simulink model "gm_sampleModel1668_5_sub_sub_sub"  (R2023a)
settings: Solver=VariableStepAuto  StartTime=0.0  StopTime=10.0  RelTol=1e-3
libraries: hdlsllib x7, simulink x1
settings Model: Creator=user1  LastModifiedBy=user1
settings OptimizationCC: BlockReduction=off  ConditionallyExecuteInputs=off
settings DebuggingCC: InheritedTsInSrcMsg=none

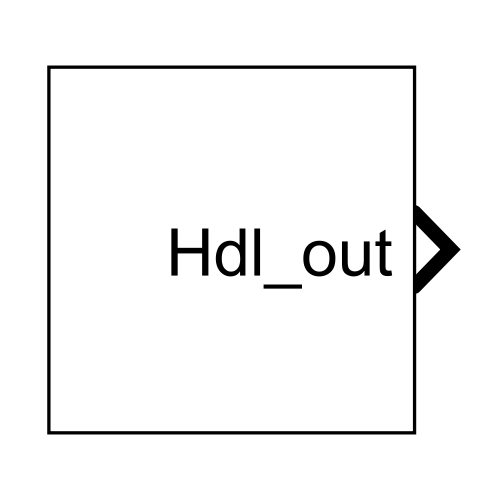
[thumbnail: Simulink's stored preview of the top-level diagram]
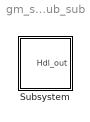
== system gm_sampleModel1668_5_sub_sub_sub ==
  Subsystem : Subsystem

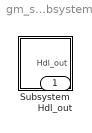
== system gm_sampleModel1668_5_sub_sub_sub/Subsystem ==
  Subsystem : Subsystem
  Hdl_out : Outport  OutDataTypeStr=uint8

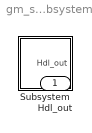
== system gm_sampleModel1668_5_sub_sub_sub/Subsystem/Subsystem ==
  Subsystem : Subsystem
  Hdl_out : Outport  OutDataTypeStr=uint8

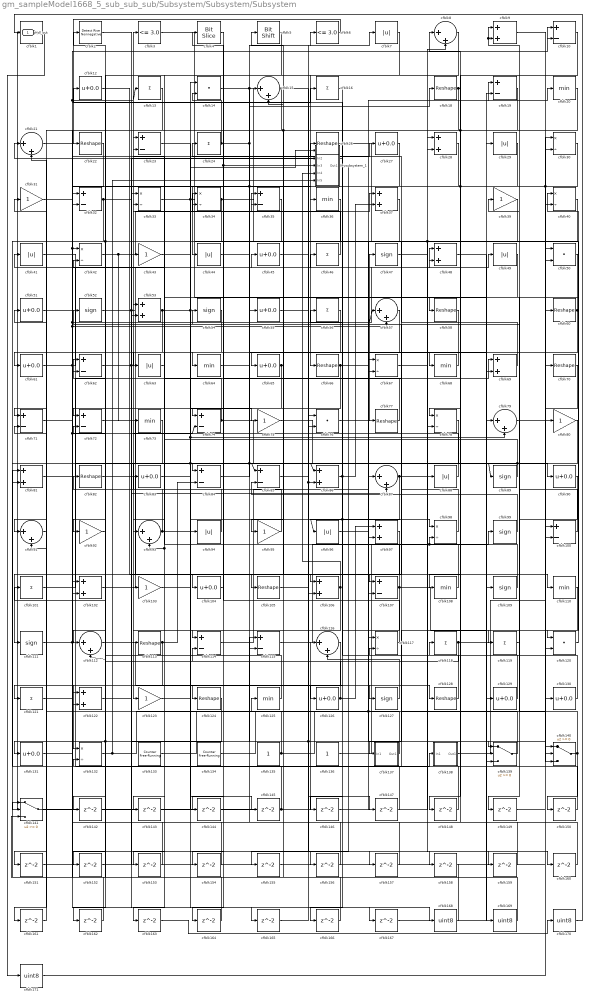
== system gm_sampleModel1668_5_sub_sub_sub/Subsystem/Subsystem/Subsystem ==
  Mysubsystem_1 : Subsystem  TreatAsAtomicUnit=on  RTWFcnName=Mysubsystem_1
      settings: RTWFcnNameOpts=User specified  RTWFileNameOpts=Use function name
  cfblk1 : simulink/Logic and Bit Operations/Bit Set  iBit=0
      settings: LibrarySourceBlock=|
      | hdlsllib/Logic and Bit
      | Operations/Bit Set
  cfblk{10,19,23,32,35,62,71..72,74,84..85,100,107,114..115} (15 alike) : Sum  Inputs=+-  OutDataTypeStr=uint8
  cfblk{13,16,24,46,56,101,118..119,121} (9 alike) : Sum  Inputs=+  OutDataTypeStr=uint8
  cfblk{9,28,37,48,53,69,81,86,97,102,106,122} (12 alike) : Sum  OutDataTypeStr=uint8
  cfblk{31,39,43,75,80,92,95,103,123} (9 alike) : Gain  OutDataTypeStr=uint8
  cfblk{12,27,45,51,55,61,65,83,90,104,126,129..131} (14 alike) : Bias  Bias=0.0  SaturateOnIntegerOverflow=off
  cfblk{18,22,26,58,60,66,70,77,82,105,113,124,128} (13 alike) : Reshape
  cfblk{20,36,64,68,73,108,110,125} (8 alike) : MinMax  OutDataTypeStr=uint8
  cfblk{47,52,54,89,99,109,111,127} (8 alike) : Signum
  cfblk{8,15,21,57,79,87,91,93,112,116} (10 alike) : Sum  Inputs=|++  OutDataTypeStr=uint8
  cfblk{30,33..34,40,42,67,78,98,117,132} (10 alike) : Product  Inputs=*/  OutDataTypeStr=uint8  RndMeth=Zero  SaturateOnIntegerOverflow=on
  cfblk{14,50,76,120} (4 alike) : DotProduct  OutDataTypeStr=uint8
  cfblk133 : hdlsllib/Sources/Counter Free-Running  NumBits=16  tsamp=-1
  cfblk134 : hdlsllib/Sources/Counter Free-Running  NumBits=16  tsamp=-1
  cfblk135 : Constant  OutDataTypeStr=uint8  SampleTime=-1
  cfblk136 : Constant  OutDataTypeStr=uint8  SampleTime=-1
  cfblk137 : Subsystem
      settings: LibrarySourceBlock=|
      | hdlsllib/Ports &
      | Subsystems/Subsystem
  cfblk138 : Subsystem
      settings: LibrarySourceBlock=|
      | hdlsllib/Ports &
      | Subsystems/Subsystem
  cfblk139 : Switch  OutDataTypeStr=uint8  SaturateOnIntegerOverflow=off  InputSameDT=off
  cfblk140 : Switch  OutDataTypeStr=uint8  SaturateOnIntegerOverflow=off  InputSameDT=off
  cfblk141 : Switch  OutDataTypeStr=uint8  SaturateOnIntegerOverflow=off  InputSameDT=off
  cfblk{142..167} (26 alike) : Delay  SampleTime=1
  cfblk{168..171} (4 alike) : DataTypeConversion  OutDataTypeStr=uint8  SaturateOnIntegerOverflow=off  RndMeth=Floor
  cfblk2 : hdlsllib/Logic and Bit Operations/Detect Rise Nonnegative  vinit=0  OutDataTypeStr=uint8
  cfblk{7,29,41,44,49,63,88,94,96} (9 alike) : Abs  OutDataTypeStr=uint8  SaturateOnIntegerOverflow=off
  cfblk3 : hdlsllib/Logic and Bit Operations/Compare To Constant  relop=<=  const=3.0  OutDataTypeStr=uint8
  cfblk4 : hdlsllib/Logic and Bit Operations/Bit Slice  lidx=7  ridx=0
  cfblk5 : hdlsllib/Logic and Bit Operations/Bit Shift  mode=Shift Left Logical  N=0
  cfblk6 : hdlsllib/Logic and Bit Operations/Compare To Constant  relop=<=  const=3.0  OutDataTypeStr=uint8
  Hdl_out : Outport  OutDataTypeStr=uint8
  wires:
  Mysubsystem_1/1(Out1) -> cfblk155/1
  cfblk171/1 -> cfblk130/1
  cfblk1/1 -> cfblk171/1
  cfblk170/1 -> cfblk1/1
  cfblk163/1 -> cfblk170/1
  cfblk169/1 -> cfblk2/1
  cfblk48/1 -> cfblk169/1
  cfblk168/1 -> cfblk51/1
  cfblk2/1 -> cfblk168/1
  cfblk167/1 -> cfblk19/2
  cfblk123/1 -> cfblk167/1
  cfblk166/1 -> cfblk15/2
  cfblk165/1 -> cfblk76/2
  cfblk164/1 -> cfblk141/1
  cfblk104/1 -> cfblk164/1
  cfblk162/1 -> cfblk122/1
  cfblk37/1 -> cfblk162/1
  cfblk161/1 -> cfblk91/2
  cfblk160/1 -> cfblk132/2
  cfblk67/1 -> cfblk160/1
  cfblk159/1 -> cfblk8/1
  cfblk158/1 -> cfblk141/3
  cfblk157/1 -> cfblk115/1
  cfblk156/1 -> cfblk35/2
  cfblk155/1 -> cfblk40/2
  cfblk154/1 -> cfblk32/1
  cfblk4/1 -> cfblk154/1
  cfblk153/1 -> cfblk62/2
  cfblk152/1 -> cfblk53/2
  cfblk151/1 -> cfblk30/2
  cfblk150/1 -> cfblk81/1
  cfblk149/1 -> cfblk120/2
  cfblk90/1 -> cfblk149/1
  cfblk148/1 -> cfblk117/2
  cfblk10/1 -> cfblk148/1
  cfblk147/1 -> cfblk71/2
  cfblk105/1 -> cfblk147/1
  cfblk146/1 -> cfblk87/1
  cfblk16/1 -> cfblk146/1
  cfblk145/1 -> cfblk33/1, Hdl_out/1
  cfblk83/1 -> cfblk145/1
  cfblk144/1 -> cfblk28/2
  cfblk143/1 -> cfblk14/1
  cfblk54/1 -> cfblk143/1
  cfblk142/1 -> cfblk107/2
  cfblk50/1 -> cfblk119/1
  cfblk56/1 -> cfblk61/1
  cfblk137/1(Out1) -> cfblk21/2
  cfblk66/1 -> cfblk122/2, cfblk139/1
  cfblk99/1 -> cfblk85/2
  cfblk47/1 -> cfblk28/1
  cfblk32/1 -> cfblk83/1, cfblk81/2
  cfblk87/1 -> cfblk106/1, cfblk20/1
  cfblk64/1 -> cfblk6/1
  cfblk70/1 -> cfblk140/2
  cfblk80/1 -> cfblk124/1
  cfblk40/1 -> cfblk86/2, cfblk106/2, cfblk78/2
  cfblk124/1 -> cfblk151/1, cfblk152/1
  cfblk60/1 -> cfblk58/1, cfblk93/1
  cfblk94/1 -> cfblk23/1
  cfblk118/1 -> cfblk60/1, cfblk114/2
  cfblk111/1 -> cfblk49/1, cfblk157/1
  cfblk84/1 -> cfblk55/1
  cfblk121/1 -> cfblk102/1
  cfblk127/1 -> cfblk116/2
  cfblk141/1 -> cfblk116/1
  cfblk43/1 -> cfblk94/1
  cfblk24/1 -> cfblk127/1, cfblk89/1, cfblk18/1, cfblk14/2
  cfblk57/1 -> cfblk105/1
  cfblk139/1 -> cfblk67/2
  cfblk65/1 -> cfblk5/1, cfblk163/1
  cfblk9/1 -> cfblk80/1
  cfblk130/1 -> cfblk118/1
  cfblk68/1 -> cfblk64/1
  cfblk125/1 -> cfblk101/1
  cfblk49/1 -> cfblk63/1
  cfblk107/1 -> cfblk35/1, cfblk129/1, cfblk166/1
  cfblk122/1 -> cfblk87/2
  cfblk103/1 -> cfblk79/2, cfblk37/1
  cfblk79/1 -> cfblk30/1
  cfblk7/1 -> cfblk103/1
  cfblk134/1 -> cfblk67/1
  cfblk35/1 -> cfblk91/1, cfblk112/2
  cfblk109/1 -> Mysubsystem_1/3(In3), cfblk4/1
  cfblk110/1 -> cfblk137/1(In1)
  cfblk96/1 -> cfblk19/1
  cfblk131/1 -> cfblk16/1, cfblk57/1
  cfblk115/1 -> cfblk79/1
  cfblk42/1 -> cfblk15/1, cfblk73/1
  cfblk55/1 -> cfblk7/1
  cfblk15/1 -> cfblk76/1, cfblk72/1
  cfblk62/1 -> Mysubsystem_1/2(In2), cfblk29/1, cfblk158/1
  cfblk34/1 -> cfblk88/1, cfblk161/1
  cfblk129/1 -> cfblk21/1
  cfblk5/1 -> cfblk112/1
  cfblk27/1 -> cfblk95/1
  cfblk29/1 -> cfblk115/2, cfblk142/1
  cfblk132/1 -> Mysubsystem_1/5(In5), cfblk8/2
  cfblk117/1 -> cfblk34/2
  cfblk88/1 -> cfblk53/1
  cfblk46/1 -> cfblk33/2
  cfblk36/1 -> cfblk114/1
  cfblk81/1 -> cfblk13/1, cfblk10/1, cfblk57/2, cfblk74/2
  cfblk71/1 -> cfblk42/1, cfblk10/2
  cfblk91/1 -> cfblk31/1
  cfblk75/1 -> cfblk140/1
  cfblk63/1 -> cfblk93/2, cfblk153/1
  cfblk33/1 -> cfblk117/1, cfblk75/1
  cfblk21/1 -> cfblk36/1
  cfblk78/1 -> cfblk141/2
  cfblk138/1(Out1) -> cfblk70/1
  cfblk98/1 -> cfblk52/1
  cfblk140/1 -> cfblk9/1, cfblk9/2, cfblk150/1
  cfblk44/1 -> cfblk69/2
  cfblk20/1 -> cfblk65/1, cfblk74/1
  cfblk18/1 -> cfblk78/1, cfblk102/2
  cfblk100/1 -> cfblk39/1
  cfblk77/1 -> cfblk34/1
  cfblk106/1 -> Mysubsystem_1/4(In4), cfblk113/1
  cfblk97/1 -> cfblk111/1
  cfblk58/1 -> cfblk96/1, cfblk126/1
  cfblk85/1 -> cfblk27/1
  cfblk53/1 -> Mysubsystem_1/1(In1), cfblk98/1, cfblk92/1
  cfblk28/1 -> cfblk44/1
  cfblk22/1 -> cfblk32/2
  cfblk112/1 -> cfblk128/1
  cfblk114/1 -> cfblk48/2
  cfblk31/1 -> cfblk26/1
  cfblk89/1 -> cfblk86/1, cfblk23/2
  cfblk23/1 -> cfblk85/1, cfblk97/2
  cfblk120/1 -> cfblk40/1
  cfblk69/1 -> cfblk24/1
  cfblk3/1 -> cfblk109/1
  cfblk86/1 -> cfblk56/1, cfblk37/2
  cfblk92/1 -> cfblk62/1
  cfblk41/1 -> cfblk100/2
  cfblk76/1 -> cfblk47/1
  cfblk14/1 -> cfblk100/1, cfblk139/3
  cfblk102/1 -> cfblk46/1
  cfblk113/1 -> cfblk121/1, cfblk84/2
  cfblk13/1 -> cfblk131/1
  cfblk8/1 -> cfblk66/1
  cfblk82/1 -> cfblk110/1
  cfblk72/1 -> cfblk84/1
  cfblk95/1 -> cfblk82/1
  cfblk19/1 -> cfblk71/1, cfblk108/1
  cfblk52/1 -> cfblk45/1, cfblk139/2
  cfblk39/1 -> cfblk107/1
  cfblk45/1 -> cfblk140/3, cfblk159/1
  cfblk30/1 -> cfblk68/1, cfblk144/1, cfblk50/2
  cfblk108/1 -> cfblk41/1, cfblk98/2
  cfblk133/1 -> cfblk125/1
  cfblk128/1 -> cfblk12/1
  cfblk73/1 -> cfblk123/1
  cfblk61/1 -> cfblk48/1, cfblk165/1
  cfblk26/1 -> cfblk120/1
  cfblk126/1 -> cfblk97/1, cfblk42/2
  cfblk135/1 -> cfblk50/1, cfblk77/1, cfblk72/2
  cfblk6/1 -> cfblk22/1
  cfblk74/1 -> cfblk90/1, cfblk43/1
  cfblk116/1 -> cfblk132/1
  cfblk101/1 -> cfblk69/1
  cfblk12/1 -> cfblk104/1
  cfblk51/1 -> cfblk138/1(In1)
  cfblk93/1 -> cfblk3/1, cfblk156/1
  cfblk119/1 -> cfblk54/1
  cfblk136/1 -> cfblk99/1

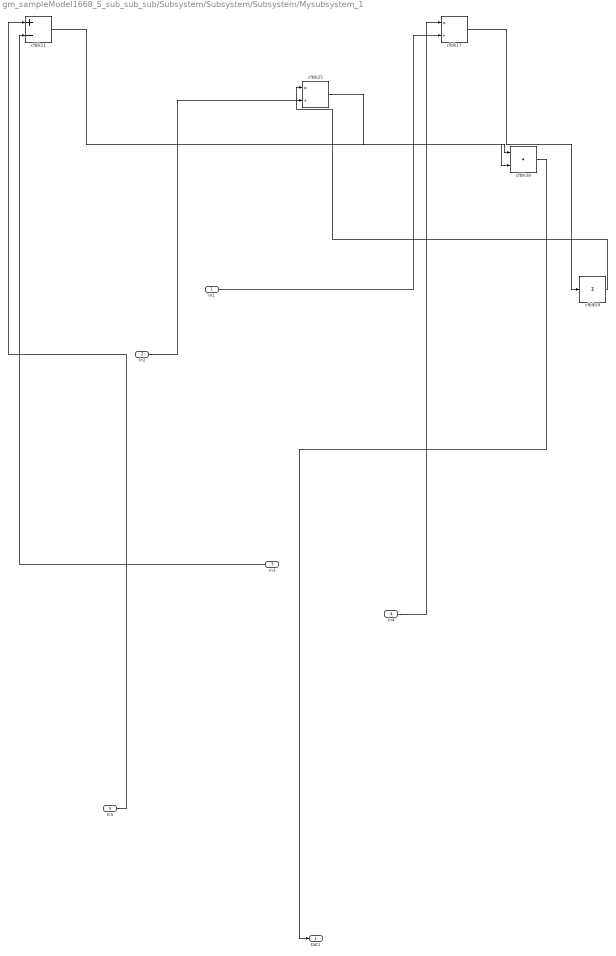
== system gm_sampleModel1668_5_sub_sub_sub/Subsystem/Subsystem/Subsystem/Mysubsystem_1 ==
  In1 : Inport
  In2 : Inport  Port=2
  In3 : Inport  Port=3
  In4 : Inport  Port=4
  In5 : Inport  Port=5
  cfblk11 : Sum  Inputs=+-
  cfblk17 : Product  Inputs=*/  RndMeth=Zero  SaturateOnIntegerOverflow=on
  cfblk25 : Product  Inputs=*/  RndMeth=Zero  SaturateOnIntegerOverflow=on
  cfblk38 : DotProduct  OutDataTypeStr=Inherit: Inherit via internal rule
  cfblk59 : Sum  Inputs=+
  Out1 : Outport
  wires:
  cfblk38/1 -> Out1/1
  In2/1 -> cfblk25/2
  cfblk17/1 -> cfblk59/1
  cfblk11/1 -> cfblk38/1
  In4/1 -> cfblk17/1
  cfblk25/1 -> cfblk38/2
  cfblk59/1 -> cfblk25/1
  In3/1 -> cfblk11/2
  In1/1 -> cfblk17/2
  In5/1 -> cfblk11/1

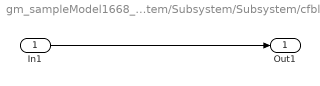
== system gm_sampleModel1668_5_sub_sub_sub/Subsystem/Subsystem/Subsystem/cfblk137 ==
  In1 : Inport
  Out1 : Outport
  wires:
  In1/1 -> Out1/1

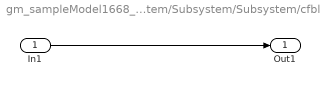
== system gm_sampleModel1668_5_sub_sub_sub/Subsystem/Subsystem/Subsystem/cfblk138 ==
  In1 : Inport
  Out1 : Outport
  wires:
  In1/1 -> Out1/1
